simulink model "OPEN_LOOP_PROCESS"  (R2024a)
settings: Solver=VariableStepAuto  StartTime=0.0  StopTime=600  RelTol=1e-3
libraries: simulink_extras x1, realtime_pacer_lib x1
settings Model: Creator=rabai  LastModifiedBy=rabai
settings RTWCC: GPUComputeCapability=3.5

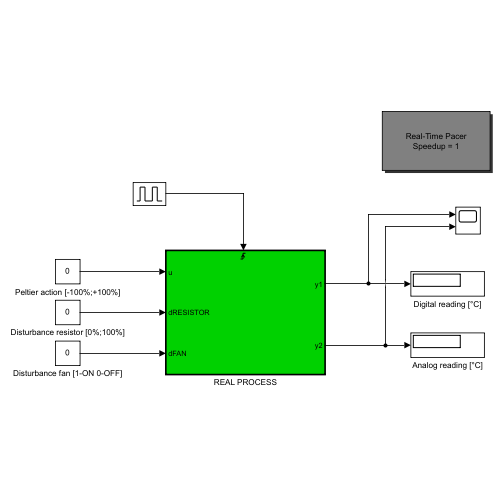
[thumbnail: Simulink's stored preview of the top-level diagram]
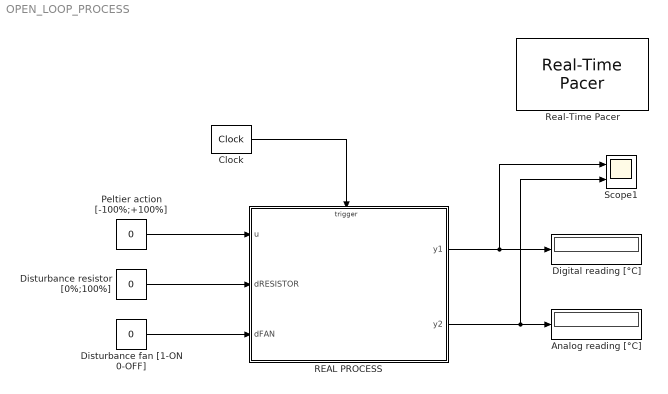
== system OPEN_LOOP_PROCESS ==
  Analog reading [°C] : Display
  Clock : simulink_extras/Flip Flops/Clock  period=1
  Digital reading [°C] : Display
  Disturbance fan [1-ON 0-OFF] : Constant  Value=0
  Disturbance resistor [0%;100%] : Constant  Value=0
  Peltier action [-100%;+100%] : Constant  Value=0
  REAL PROCESS : Subsystem
  Real-Time Pacer : realtime_pacer_lib/Real-Time Pacer  simTimePerRealTime=1
      settings: SourceProductName=Real-Time Pacer
  Scope1 : Scope  NumInputPorts=2
  wires:
  Clock/1 -> REAL PROCESS/Trigger
  Peltier action [-100%;+100%]/1 -> REAL PROCESS/1(u)
  Disturbance fan [1-ON 0-OFF]/1 -> REAL PROCESS/3(dFAN)
  Disturbance resistor [0%;100%]/1 -> REAL PROCESS/2(dRESISTOR)
  REAL PROCESS/1(y1) -> Digital reading [°C]/1, Scope1/1
  REAL PROCESS/2(y2) -> Analog reading [°C]/1, Scope1/2

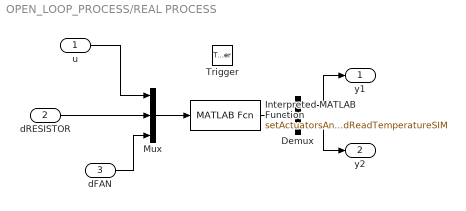
== system OPEN_LOOP_PROCESS/REAL PROCESS ==
  u : Inport
  dRESISTOR : Inport  Port=2
  dFAN : Inport  Port=3
  Trigger : TriggerPort  VariantControl=(inherit)  PortDimensions=1
  Demux : Demux  Outputs=2
  Interpreted MATLAB Function : MATLABFcn  MATLABFcn=setActuatorsAndReadTemperatureSIM  OutputDimensions=2
  Mux : Mux  Inputs=3
  y1 : Outport
  y2 : Outport  Port=2
  wires:
  Interpreted MATLAB Function/1 -> Demux/1
  Demux/1 -> y1/1
  Demux/2 -> y2/1
  u/1 -> Mux/1
  dRESISTOR/1 -> Mux/2
  dFAN/1 -> Mux/3
  Mux/1 -> Interpreted MATLAB Function/1
